simulink model "rom1"  (Simulink 7.6)
settings: Solver=FixedStepDiscrete  StartTime=0.0  StopTime=1  FixedStep=1  RelTol=1e-3
libraries: simulink x10
settings Model: Creator=jordan  LastModifiedBy=jordan
settings DataIOCC: LimitDataPoints=off  SaveOutput=off  SignalLogging=off  DSMLogging=off  SaveTime=off
settings OptimizationCC: BlockReduction=off  ConditionallyExecuteInputs=off  InlineParams=on

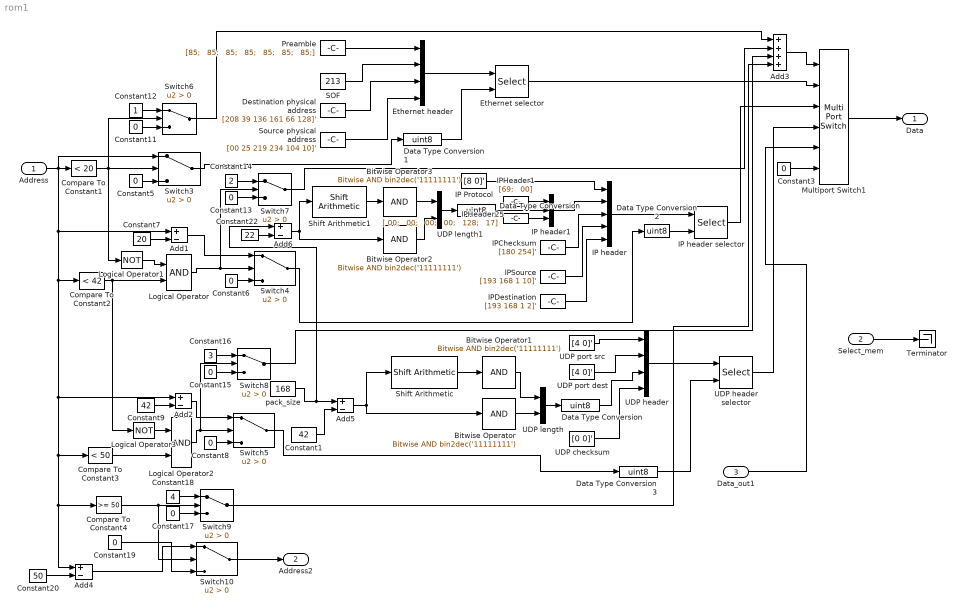
== system rom1 ==
  Address : Inport  OutDataTypeStr=fixdt(0,11,0)
  Select_mem : Inport  Port=2  OutDataTypeStr=fixdt(0,4,0)
  Data_out1 : Inport  Port=3  OutDataTypeStr=uint8
  Add1 : Sum  Inputs=+-
  Add2 : Sum  Inputs=+-
  Add3 : Sum  Inputs=++++
  Add4 : Sum  Inputs=+-  AccumDataTypeStr=fixdt(0,14,0)  OutDataTypeStr=fixdt(0,14,0)
  Add5 : Sum  Inputs=+-  OutDataTypeStr=uint16
  Add6 : Sum  Inputs=+-  OutDataTypeStr=uint16
  Bitwise Operator{,1..3} (4 alike) : simulink/Logic and Bit Operations/Bitwise Operator  logicop=AND  UseBitMask=on  BitMask=bin2dec('11111111')  BitMaskRealWorld=Stored Integer
  Compare To Constant1 : simulink/Logic and Bit Operations/Compare To Constant  SystemSampleTime=-1  relop=<  const=20  LogicOutDataTypeMode=boolean
  Compare To Constant2 : simulink/Logic and Bit Operations/Compare To Constant  SystemSampleTime=-1  relop=<  const=42  LogicOutDataTypeMode=boolean
  Compare To Constant3 : simulink/Logic and Bit Operations/Compare To Constant  SystemSampleTime=-1  relop=<  const=50  LogicOutDataTypeMode=boolean
  Compare To Constant4 : simulink/Logic and Bit Operations/Compare To Constant  SystemSampleTime=-1  relop=>=  const=50  LogicOutDataTypeMode=boolean
  Constant1 : Constant  Value=42  OutDataTypeStr=uint8
  Constant{3,5..6,8,11,13,15,17} (8 alike) : Constant  Value=0  OutDataTypeStr=uint8
  Constant12 : Constant  OutDataTypeStr=uint8
  Constant14 : Constant  Value=2  OutDataTypeStr=uint8
  Constant16 : Constant  Value=3  OutDataTypeStr=uint8
  Constant18 : Constant  Value=4  OutDataTypeStr=uint8
  Constant19 : Constant  Value=0  OutDataTypeStr=fixdt(0,14,0)
  Constant20 : Constant  Value=50  OutDataTypeStr=uint8
  Constant22 : Constant  Value=22  OutDataTypeStr=uint8
  Constant7 : Constant  Value=20  OutDataTypeStr=uint8
  Constant9 : Constant  Value=42  OutDataTypeStr=uint8
  Data Type Conversion{,1..3,5} (5 alike) : DataTypeConversion  OutDataTypeStr=uint8
  "Destination physical address " : Constant  Value=[208 39 136 161 66 128]'  OutDataTypeStr=uint8
  Ethernet header : Mux
  Ethernet selector : Selector  IndexMode=Zero-based  InputPortWidth=20  IndexOptions=Index vector (port)  Indices=[1 3]  OutputSizes=1
  IP Protocol : Constant  Value=[8 0]'  OutDataTypeStr=uint8
  IP header : Mux  Inputs=5
  IP header selector : Selector  IndexMode=Zero-based  InputPortWidth=22  IndexOptions=Index vector (port)  Indices=[1 3]  OutputSizes=1
  IP header1 : Mux  Inputs=3
  IPChecksum : Constant  Value=[180 254]'  OutDataTypeStr=uint8
  IPDestination : Constant  Value=[193 168 1 2]'  OutDataTypeStr=uint8
  IPHeader1 : Constant  Value=|  OutDataTypeStr=uint8
      | [69;
      |   00]
  IPHeader2 : Constant  Value=|  OutDataTypeStr=uint8
      | [ 00;
      |   00;
      |   00;
      |   00;
      |   128;
      |   17]
  IPSource : Constant  Value=[193 168 1 10]'  OutDataTypeStr=uint8
  Logical Operator : Logic  AllPortsSameDT=off  OutDataTypeStr=boolean
  Logical Operator1 : Logic  Operator=NOT  AllPortsSameDT=off  OutDataTypeStr=boolean
  Logical Operator2 : Logic  AllPortsSameDT=off  OutDataTypeStr=boolean
  Logical Operator3 : Logic  Operator=NOT  AllPortsSameDT=off  OutDataTypeStr=boolean
  Multiport Switch1 : MultiPortSwitch  Inputs=4  DataPortForDefault=Additional data port  DiagnosticForDefault=None  zeroidx=off
  Preamble : Constant  Value=|  OutDataTypeStr=uint8
      | [85;
      |   85;
      |   85;
      |   85;
      |   85;
      |   85;
      |   85;]
  SOF : Constant  Value=213  OutDataTypeStr=uint8
  Shift Arithmetic : simulink/Logic and Bit Operations/Shift Arithmetic  SystemSampleTime=-1  nBitShiftRight=8  nBinPtShiftRight=0
  Shift Arithmetic1 : simulink/Logic and Bit Operations/Shift Arithmetic  SystemSampleTime=-1  nBitShiftRight=8  nBinPtShiftRight=0
  Source physical address : Constant  Value=[00 25 219 234 104 10]'  OutDataTypeStr=uint8
  Switch{3..10} (8 alike) : Switch  Criteria=u2 > Threshold
  Terminator : Terminator
  UDP checksum : Constant  Value=[0 0]'  OutDataTypeStr=uint8
  UDP header : Mux
  UDP header selector : Selector  IndexMode=Zero-based  InputPortWidth=8  IndexOptions=Index vector (port)  Indices=[1 3]  OutputSizes=1
  UDP length : Mux  Inputs=2
  UDP length1 : Mux  Inputs=2
  UDP port dest : Constant  Value=[4 0]'  OutDataTypeStr=uint8
  UDP port src : Constant  Value=[4 0]'  OutDataTypeStr=uint8
  pack_size : Constant  Value=168  OutDataTypeStr=uint8
  Data : Outport  OutDataTypeStr=uint8  InitialOutput=0
  Address2 : Outport  Port=2  OutDataTypeStr=fixdt(0,14,0)
  wires:
  Address/1 -> Compare To Constant1/1, Switch3/1, Add1/1, Add2/1, Compare To Constant3/1, Compare To Constant4/1, Add4/1, Compare To Constant2/1
  Multiport Switch1/1 -> Data/1
  Preamble/1 -> Ethernet header/1
  SOF/1 -> Ethernet header/2
  "Destination physical address "/1 -> Ethernet header/3
  Source physical address/1 -> Ethernet header/4
  Ethernet header/1 -> Ethernet selector/1
  Ethernet selector/1 -> Multiport Switch1/2
  IP Protocol/1 -> IP header/1
  IPChecksum/1 -> IP header/3
  IPSource/1 -> IP header/4
  IPDestination/1 -> IP header/5
  IP header/1 -> IP header selector/1
  IP header selector/1 -> Multiport Switch1/3
  Constant3/1 -> Multiport Switch1/6
  UDP port src/1 -> UDP header/1
  UDP port dest/1 -> UDP header/2
  UDP length/1 -> Data Type Conversion/1
  UDP checksum/1 -> UDP header/4
  pack_size/1 -> Add5/1, Add6/1
  Bitwise Operator/1 -> UDP length/2
  Bitwise Operator1/1 -> UDP length/1
  Shift Arithmetic/1 -> Bitwise Operator1/1
  Data Type Conversion/1 -> UDP header/3
  UDP header/1 -> UDP header selector/1
  UDP header selector/1 -> Multiport Switch1/4
  Compare To Constant1/1 -> Switch6/2, Logical Operator1/1, Switch3/2
  Constant5/1 -> Switch3/3
  Switch3/1 -> Data Type Conversion1/1
  Compare To Constant2/1 -> Logical Operator/2, Logical Operator3/1
  Logical Operator1/1 -> Logical Operator/1
  Constant6/1 -> Switch4/3
  Logical Operator/1 -> Switch4/2, Switch7/2
  Switch4/1 -> Data Type Conversion2/1
  Constant7/1 -> Add1/2
  Add1/1 -> Switch4/1
  Logical Operator3/1 -> Logical Operator2/1
  Logical Operator2/1 -> Switch5/2, Switch8/2
  Compare To Constant3/1 -> Logical Operator2/2
  Constant8/1 -> Switch5/3
  Constant9/1 -> Add2/2
  Add2/1 -> Switch5/1
  Switch5/1 -> Data Type Conversion3/1
  Constant11/1 -> Switch6/3
  Constant12/1 -> Switch6/1
  Switch6/1 -> Add3/1
  Constant13/1 -> Switch7/3
  Constant14/1 -> Switch7/1
  Add3/1 -> Multiport Switch1/1
  Switch7/1 -> Add3/2
  Constant15/1 -> Switch8/3
  Constant16/1 -> Switch8/1
  Switch8/1 -> Add3/3
  Constant17/1 -> Switch9/3
  Constant18/1 -> Switch9/1
  Switch9/1 -> Add3/4
  Constant19/1 -> Switch10/3
  Constant20/1 -> Add4/2
  Add4/1 -> Switch10/1
  Select_mem/1 -> Terminator/1
  Switch10/1 -> Address2/1
  Data Type Conversion1/1 -> Ethernet selector/2
  Data Type Conversion2/1 -> IP header selector/2
  Data Type Conversion3/1 -> UDP header selector/2
  Constant1/1 -> Add5/2
  Add5/1 -> Shift Arithmetic/1, Bitwise Operator/1
  Compare To Constant4/1 -> Switch9/2, Switch10/2
  IP header1/1 -> IP header/2
  IPHeader1/1 -> IP header1/1
  IPHeader2/1 -> IP header1/3
  Data Type Conversion5/1 -> IP header1/2
  UDP length1/1 -> Data Type Conversion5/1
  Bitwise Operator2/1 -> UDP length1/2
  Bitwise Operator3/1 -> UDP length1/1
  Shift Arithmetic1/1 -> Bitwise Operator3/1
  Constant22/1 -> Add6/2
  Add6/1 -> Bitwise Operator2/1, Shift Arithmetic1/1
  Data_out1/1 -> Multiport Switch1/5
